simulink model "Multibody_Pull"  (R2022b)
settings: Solver=VariableStepAuto  StartTime=0.0  StopTime=10.0  RelTol=1e-3  AbsTol=1e-3  EnableMultiTasking=on
libraries: sm_lib x3, nesl_utility x1
settings Model: Creator=david  LastModifiedBy=david
settings SolverCC: AutoScaleAbsTol=off  AlgebraicLoopSolver=TrustRegion  MaxZcPerStep=1
settings DataIOCC: LimitDataPoints=on  MaxDataPoints=10000
settings OptimizationCC: LifeSpan=inf
settings DebuggingCC: UnconnectedInputMsg=warning  UnconnectedOutputMsg=warning  UnconnectedLineMsg=warning  AllowSymbolicDim=off  SFUnexpectedBacktrackingDiag=warning  SFNoUnconditionalDefaultTransitionDiag=warning  SFExecutionAtInitializationDiag=none  SFMachineParentedDataDiag=warning  ArithmeticOperatorsInVariantConditions=warning
settings ModelReferenceCC: EnableRefExpFcnMdlSchedulingChecks=on
settings SFSimCC: SimUseLocalCustomCode=off  CustomCodeUndefinedFunction=UseInterfaceOnly
settings RTWCC: RTWUseLocalCustomCode=off  DLArmComputeVersion=19.05
settings CodeAppCC: StateflowObjectComments=on
settings GRTTargetCC: TargetLangStandard=C89/C90 (ANSI)
settings ConfigComp: CovMetricSettings=dw  CovSaveCumulativeToWorkspaceVar=on  CovSaveSingleToWorkspaceVar=on  CovExternalEMLEnable=off  CovSFcnEnable=off
settings SimscapeCC: SimscapeLogType=all  SimscapeLogSimulationStatistics=on  SimscapeLogDataHistory=10000

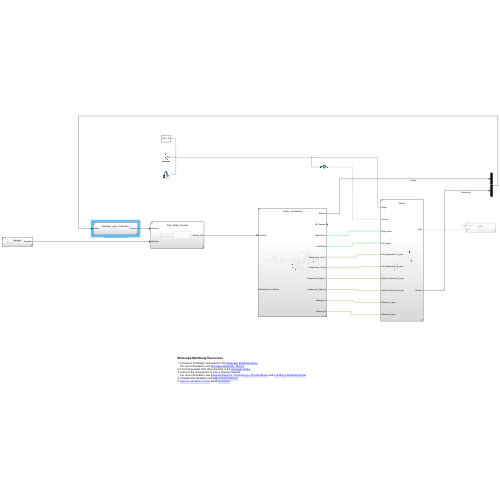
[thumbnail: Simulink's stored preview of the top-level diagram]
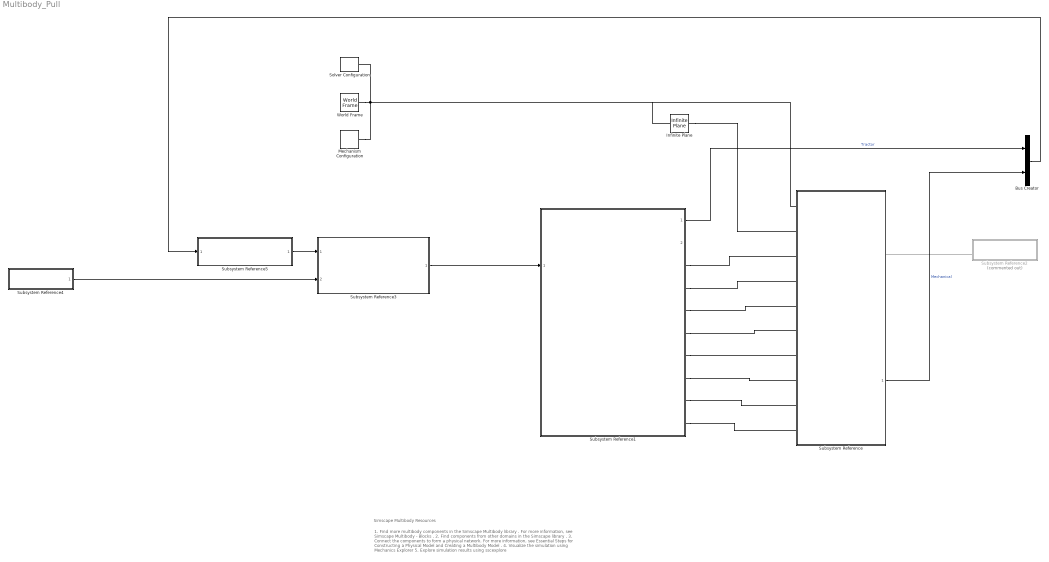
== system Multibody_Pull ==
  note: 1. Find more multibody components in the Simscape Multibody library .
      | For more information, see Simscape Multibody - Blocks .
      | 2. Find components from other domains in the Simscape library .
      | 3. Connect the components to form a physical network.
      | For more information, see Essential Steps for Constructing a Physical Model and Creating a Multibody Model .
      | 4. Visualize the simulation using Mechanics Explorer
      | 5. Explore simulation results using sscexplore
  note: Simscape Multibody Resources
  Bus Creator : BusCreator  Inputs=2
  Infinite Plane : sm_lib/Curves and Surfaces/Infinite Plane  GraphicType=Rectangle  GraphicPlaneWidth=10  GraphicPlaneWidthUnits=m  GraphicPlaneHeight=10  GraphicPlaneHeightUnits=m  GraphicVisPropType=SimpleVisualProperties  GraphicDiffuseColor=[0.5 0.5 0.5]  GraphicOpacity=0.25  GraphicSpecularColor=[0.5 0.5 0.5 1.0]  GraphicAmbientColor=[0.15 0.15 0.15 1.0]  GraphicEmissiveColor=[0.0 0.0 0.0 1.0]  GraphicShininess=75
  Mechanism Configuration : sm_lib/Utilities/Mechanism Configuration  UniformGravity=Constant  GravityVector=[0 0 -9.80665]  GravityUnits=m/s^2  LinearizationDelta=0.001  JointModeTransitionNonlinearIterations=2
  Solver Configuration : nesl_utility/Solver Configuration  PhysicalDomain=network_engine_domain  SubClassName=solver  LeftPortType=input  RightPortType=generic  Tones=[]  Harmonics=[]  SimulateNoise=off  Profile=off  UseLocalSampling=off  EnableSwitchedLinearOptims=on  FrequencyDomain=off  UseCCode=off  RelTol=0.001  AbsTol=1e-06  MinStep=1e-09  ToWorkspace=off  RevertToSquareIcSolve=off  NumHomotopyIterations=100  PhasorMode=off  PhasorModeNumHarmonics=1  ConsistencySolver=NEWTON_XTOL_AFTER_FTOL  IndexReductionMethod=DerivativeReplacement  DoDC=off  ResidualTolerance=1e-09  ConsistencyTolSource=GLOBAL  ConsistencyAbsTol=0.001  ConsistencyRelTol=0.001  ConsistencyTolFactor=0.001  UseLocalSolver=off  LocalSolverChoice=NE_BACKWARD_EULER_ADVANCER  ResolveIndetEquations=on  FunctionEvalNumThread=1  LocalSolverSampleTime=0.001  DoFixedCost=off  MaxNonlinIter=3  MaxModeIter=2  ComputeImpulses=off  ImpulseIterations=2  LinearAlgebra=Sparse  LinearAlgebraNumThread=0  EquationFormulation=NE_TIME_EF  DelaysMemoryBudget=1024  AutomaticFiltering=on  FilteringTimeConstant=0.001  PartitionStorageMethod=AS_NEEDED  PartitionMemoryBudget=1024  PartitionMethod=FAST
  Subsystem Reference : Subsystem  ReferencedSubsystem=Tractor
      settings: PortSchema="{\"entries\":[{\"content\":{\"sides\":[{\"content\":{\"connectorIds\":[\"LConn1\",\"LConn2\",\"LConn3\",\"LConn4\",\"LConn8\",\"LConn9\",\"LConn10\",\"LConn11\",\"LConn6\",\"LConn7\"]},\"type\":\"ConnectorPlacement.EquallySpacedRectSide\",\"uuid\":\"86ce24e1-0a50-42d7-a6d6-97ecfec99729\"},{\"content\":{\"connectorIds\":[\"LConn5\",\"Out1\"],\"side\":\"RIGHT\"},\"type\":\"ConnectorPlacement.EquallySpacedRectSide\",\"uuid\":\"37e84e1b-0aba-4668-bcfc-302caca33675\"},{\"content\":{\"connectorIds\":[],\"side\":\"TOP\"},\"type\":\"ConnectorPlacement.EquallySpacedRectSide\",\"uuid\":\"19e32e16-e086-493a-a7e0-dc3917c8b4c6\"}]},\"type\":\"ConnectorPlacement.EquallySpacedConnector\",\"uuid\":\"fcb69214-6329-4234-a6bc-b065e70085cc\"}],\"packageUris\":[\"http://schema.mathworks.com/mf0/Connector/R2020b\"],\"version\":\"1.0\"}"
  Subsystem Reference1 : Subsystem  ReferencedSubsystem=Tractor_mechanical
      settings: PortSchema="{\"entries\":[{\"content\":{\"sides\":[{\"content\":{\"connectorIds\":[\"In1\",\"LConn1\"]},\"type\":\"ConnectorPlacement.EquallySpacedRectSide\",\"uuid\":\"7f8cd349-61d0-4407-9fae-99dbb21d5e73\"},{\"content\":{\"connectorIds\":[\"Out1\",\"Out2\",\"RConn2\",\"RConn1\",\"RConn3\",\"RConn4\",\"RConn5\",\"RConn6\",\"RConn7\",\"RConn8\"],\"side\":\"RIGHT\"},\"type\":\"ConnectorPlacement.EquallySpacedRectSide\",\"uuid\":\"ec88d6fe-5f90-4ad5-a75d-cd981446d315\"},{\"content\":{\"connectorIds\":[],\"side\":\"TOP\"},\"type\":\"ConnectorPlacement.EquallySpacedRectSide\",\"uuid\":\"cb74be0e-c61b-48e1-916d-6b4f302a841f\"}]},\"type\":\"ConnectorPlacement.EquallySpacedConnector\",\"uuid\":\"2b28b40f-44cc-42f8-aac3-ff97f91fdd0a\"}],\"packageUris\":[\"http://schema.mathworks.com/mf0/Connector/R2020b\"],\"version\":\"1.0\"}"
  Subsystem Reference2 : Subsystem  Commented=on  ReferencedSubsystem=Sled
      settings: PortSchema="{\"entries\":[{\"content\":{\"sides\":[{\"content\":{\"connectorIds\":[\"LConn2\",\"LConn1\"]},\"type\":\"ConnectorPlacement.EquallySpacedRectSide\",\"uuid\":\"4ef1d177-4f4c-4c27-ada6-f46ac747013f\"},{\"content\":{\"connectorIds\":[],\"side\":\"RIGHT\"},\"type\":\"ConnectorPlacement.EquallySpacedRectSide\",\"uuid\":\"5ab6b5fb-6a8a-4c2b-be95-2ba50a0bdbaa\"},{\"content\":{\"connectorIds\":[],\"side\":\"TOP\"},\"type\":\"ConnectorPlacement.EquallySpacedRectSide\",\"uuid\":\"70193827-c960-4a8f-ada4-d8e41c7f67e3\"}]},\"type\":\"ConnectorPlacement.EquallySpacedConnector\",\"uuid\":\"352b12dc-3589-437e-8b91-791fe864bbd0\"}],\"packageUris\":[\"http://schema.mathworks.com/mf0/Connector/R2020b\"],\"version\":\"1.0\"}"
  Subsystem Reference3 : Subsystem  ReferencedSubsystem=Plant_Model_Controls
  Subsystem Reference4 : Subsystem  ReferencedSubsystem=Operator
  Subsystem Reference5 : Subsystem  ReferencedSubsystem=Multibody_Input_Calibration
  World Frame : sm_lib/Frames and Transforms/World Frame
  wires:
  Subsystem Reference3/1 -> Subsystem Reference1/1
  Subsystem Reference4/1 -> Subsystem Reference3/2
  Bus Creator/1 -> Subsystem Reference5/1
  Subsystem Reference/1 -> Bus Creator/2  "Mechanical"
  Subsystem Reference1/1 -> Bus Creator/1  "Tractor"
  Subsystem Reference5/1 -> Subsystem Reference3/1
  connections:
  World Frame/RConn1 -- Infinite Plane/LConn1 -- Subsystem Reference/LConn1 -- Mechanism Configuration/RConn1 -- Solver Configuration/RConn1
  Subsystem Reference1/RConn1 -- Subsystem Reference/LConn4
  Subsystem Reference1/RConn2 -- Subsystem Reference/LConn3
  Subsystem Reference1/RConn3 -- Subsystem Reference/LConn8
  Subsystem Reference1/RConn4 -- Subsystem Reference/LConn9
  Subsystem Reference1/RConn5 -- Subsystem Reference/LConn10
  Subsystem Reference1/RConn6 -- Subsystem Reference/LConn11
  Subsystem Reference1/RConn7 -- Subsystem Reference/LConn6
  Subsystem Reference1/RConn8 -- Subsystem Reference/LConn7
  Subsystem Reference2/LConn1 -- Subsystem Reference/LConn5
  Infinite Plane/RConn1 -- Subsystem Reference/LConn2
